simulink model "ADCS_Simulink"  (R2025b)
settings: Solver=FixedStepAuto  StartTime=0  StopTime=30  FixedStep=0.001  RelTol=1e-3
PreLoadFcn:
  | addpath(genpath('../'))
undefined symbols (not defined in the file or in its folder): DiscIntNeverNeededParam, IAU, juliandate
libraries: vrlib x16, simulink_extras x7, sharedtransform x5, sharedutil x4, aerolibutil x4, sFunctionLibrary x4, simulink x2, matrix_library x2, aerolibtransform2 x2
(part 2 of 2)

== matlab function ADCS_Simulink/Simulate Omega Rates/Wheel Torque ==
  data: wheel_speeds input; mag_bf input; GsValues input; L_R input; us output; tauMTB output; t_3axis output
function [us, tauMTB,t_3axis]  = f(wheel_speeds, mag_bf, GsValues, L_R)
% MATLAB Function block version of WheelTorque_Command
%
% Inputs:
%   wheel_speeds [4x1]   : Reaction wheel speeds [rad/s]
%   mag_bf       [3x1]   : Magnetic field vector in body frame [T]
%   GsValues     [3x4]   : Wheel geometry / spin axis matrix
%   L_R_input    [3x1]   : Desired control torque from PD controller [Nm]
%
% Output:
%   out_u [7x1] : [us(4x1); tauMTB(3x1)]

    % Constants
    Iws = 0.000029382450521;   % Wheel spin axis inertia [kg·m^2]
    c   = 0.025;                % Reaction wheel torque to magtorquer scaler
    OmegaD = rpm_to_rads(250) * ones(4,1);  % Desired wheel bias [rad/s]

    % Wheel speed vector
    Omega = wheel_speeds(:);

    % L_R from PD controller
    L_R = L_R(:);

    % Torque rod transformation (identity)
    Gt = eye(3);

    % Compute pseudo-inverse of Gs
    Gs = GsValues;
    Gs_pinv = pinv(Gs);

    % RW torque required to track commanded torque
    usReq = Gs_pinv * (-L_R);  %usReq is a 4 by 1 quantity

    % Despin torque
    usStar = -c * Iws * (Omega - OmegaD);

    % Skew-symmetric matrix of magnetic field
    B_tilde = [   0      -mag_bf(3)  mag_bf(2);
               mag_bf(3)     0      -mag_bf(1);
              -mag_bf(2)  mag_bf(1)     0     ];

     
    Btilde_Gt = B_tilde * Gt;
    muStar = -pinv(Btilde_Gt) * Gs * usStar;
    for i = 1:3
        if(muStar(i)>.1)
            muStar(i) = .1;
        end
        if(muStar(i)<-.1)
            muStar(i) = -.1;
        end
    end

    % Magnetic torque
    tauMTB = -(Btilde_Gt) * muStar;

    % deltaU = pinv(Gs) * (tauMTB - Gs*usStar)
    deltaU = Gs_pinv * (tauMTB - Gs * usStar);

    % Actual applied RW torque
    us = usReq + usStar + deltaU;

    for i = 1:4
        if(us(i)>.0032)
        us(i) = .0032;
        end
        if(us(i)<-.0032)
        us(i)=-.0032;
        end
    end

    t_3axis = -Gs*us;

end

% Helper: RPM to rad/s
function rad_s = rpm_to_rads(rpm)
    rad_s = rpm * (2*pi/60);
end

== matlab function ADCS_Simulink/Single Axis Error/Compute single axis rotation ==
  data: a input; y output; b input
function y = fcn(a, b)

axis = cross(a, b);
axis_norm = norm(axis);

if axis_norm < 1e-8
    if dot(a,b) > 0   %Vectors is parallel
        y = [1; 0; 0; 0];

    else              %Vectors are antiparallel
        axis = null(a(:).');
        axis = axis(:,1)/norm(axis(:,1));
        y = [0; axis];
    end
    return
end

axis = cross(a, b);
axis_norm = norm(axis);
axis = axis / axis_norm;
angle = acos(dot(a, b) / (norm(a)*norm(b)));

y = zeros(4,1);
y(1) = cos(angle / 2);
y(2:4) = axis * sin(angle / 2);

% if(y(1)<0)
%     y=-y;
% end

== matlab function ADCS_Simulink/Estimate Attitude/QUEST/MATLAB Function1 ==
  data: B_NED input; B_ECI output; lat input; lon input; JD input
function B_ECI = ned2eci(B_NED, lat, lon, JD)
% Converts magnetic field vector from NED to ECI
% Inputs:
%   B_NED = [Bn; Be; Bd] magnetic field vector in NED [any units]
%   lat, lon = geodetic latitude, longitude [deg]
%   JD = Julian Date
% Output:
%   B_ECI = [Bx; By; Bz] in ECI coordinates [same units]

lon = deg2rad(lon);
lat = deg2rad(lat);
% ----- 1. Compute GMST -----
JD0 = floor(JD + 0.5) - 0.5;
H = (JD - JD0) * 24;             % hours since 0h UT
D = JD - 2451545.0;
D0 = JD0 - 2451545.0;
T = D / 36525;

GMST_hours = 6.697374558 + 0.06570982441908 * D0 + 1.00273790935 * H + 0.000026 * T^2;
GMST_hours = mod(GMST_hours, 24);         % wrap 0-24h
theta_g = deg2rad(15 * GMST_hours);       % convert to radians

% ----- 2. Rotation from NED -> ECEF -----
R_ECEF_NED = [ -sin(lat)*cos(lon), -sin(lat)*sin(lon),  cos(lat);
               -sin(lon),            cos(lon),           0;
               -cos(lat)*cos(lon),  -cos(lat)*sin(lon), -sin(lat) ];

% ----- 3. Rotation from ECEF -> ECI -----
R_ECI_ECEF = [ cos(theta_g), -sin(theta_g), 0;
               sin(theta_g),  cos(theta_g), 0;
               0,              0,           1 ];

% ----- 4. Combine rotations -----
B_ECI = R_ECI_ECEF * R_ECEF_NED * B_NED;
end

== matlab function ADCS_Simulink/Simulate Omega Rates/Clamp WS ==
  data: u input; y output
function y = fcn(u)

max_threshold=6500*((2*pi)/60);
min_threshold=120*((2*pi)/60);

for i=1:4
if(u(i)>max_threshold)
    u(i)=max_threshold;
elseif(u(i)<-min_threshold)
    u(i)=-min_threshold;
end

end
y=u;

== matlab function ADCS_Simulink/Create Desired Quaternion/DCOMM & CSAC/MATLAB Function ==
  data: JD_now input; day output
function day = fcn(JD_now)

baseJD_start =  2.460950250000000e+06;
day = JD_now - baseJD_start;

== matlab function ADCS_Simulink/Angle Error1 ==
  data: u input; y output
function y = fcn(u)
    a = u(1);
    
    y = 2 * acos(a);
end

== matlab function ADCS_Simulink/Create Desired Quaternion/Check Flippage ==
  data: q input; y output
function y = fcn(q)

% persistent q_prev;
% if(isempty(q_prev))
%     q_prev=q;
% end
% 
% if(dot(q_prev,q)<0)
%     q=-q;
% end
% 
% q_prev=q;
% y=q;

if(q(1)<=0)
y=-q;
else
y=q;
end
end

== matlab function ADCS_Simulink/Estimate Attitude/QUEST/Sun_vec_eci ==
  data: sun_vec_eci output; decyear output; day output; t_utc input
function [sun_vec_eci, decyear, day] = SunVecECI_codegen(t_utc)
% Codegen-safe function for Simulink
% Input: t_utc (Julian Date)
% Outputs:
%   sun_vec_eci - 3x1 Sun unit vector in ECI
%   decyear     - decimal year (for IGRF)
%   day         - day of month (for IGRF)

% --- Constants ---
JD_J2000 = 2451545.0; % reference JD for 2000-01-01 12:00 UTC

% --- Compute approximate year ---
days_since_2000 = t_utc - JD_J2000;
year = 2000 + floor(days_since_2000 / 365.25);

% --- Compute day-of-year fraction ---
JD_start_of_year = JD_J2000 + (year-2000)*365.25; % approximate start of year
frac_day_of_year = t_utc - JD_start_of_year;

% --- Compute day of month (simplified for IGRF) ---
% approximate: 12 months = 365.25/12 ~ 30.4375 days per month
day = floor(mod(frac_day_of_year, 30.4375)) + 1;

% --- Decimal year ---
decyear = year + frac_day_of_year / 365.25;

% --- Clamp for IGRF ---
if decyear > 2025
    decyear = 2025;
elseif decyear < 1900
    decyear = 1900;
end

% --- Sun vector in ECI ---
D_days = t_utc - JD_J2000; % days since J2000
g = 357.529 + 0.98560028 * D_days;           
q = 280.459 + 0.98564736 * D_days;          
L = q + 1.914666471*sind(g) + 0.018994643*sind(2*g);
e = 23.439291 - 0.0130042*(D_days/36525); 

x = cosd(L);
y = cosd(e)*sind(L);
z = sind(e)*sind(L);
 sun_vec_eci = [x; y; z];
% sun_vec_eci= [-0.9672; 4; -0.10];

end

== matlab function ADCS_Simulink/Estimate Attitude/QUEST/Trace ==
  data: x input; y output
function y = fcn(x)

y=x(1,1)+x(2,2)+x(3,3);

== matlab function ADCS_Simulink/Angle Error2 ==
  data: u input; y output
function y = fcn(u)
    a = u(1);
    
    y = 2 * acos(a);
end

== matlab function ADCS_Simulink/Estimate Attitude/buildBk ==
  data: magVec input single; y output single size=[3 2]; sunVec input single
function y = combineMagSunMeas(magVec,sunVec)
    
    y = single(zeros(3,2));
    y(:,1) = magVec;
    y(:,2) = sunVec;
end

== matlab function ADCS_Simulink/Estimate Attitude/buildEci_k ==
  data: magVec input single; y output single size=[3 2]; sunVec input single
function y = combineMagSunMeas(magVec,sunVec)
    
    y = single(zeros(3,2));
    y(:,1) = magVec;
    y(:,2) = sunVec;
end

== matlab function ADCS_Simulink/Estimate Attitude/Angle Error2 ==
  data: u input; y output
function y = fcn(u)
    a = u(1);
    
    y = 2 * acos(a);
end

== matlab function ADCS_Simulink/Estimate Attitude/Check Flippage ==
  data: u input; y output
function y = fcn(u)

if u(1)<0
     y = -u;
else 
    y=u;
end

== matlab function ADCS_Simulink/Create Desired Quaternion/create DCM ==
  data: y output; dv input; v1 output; v2 output; vel input; doter output; var output
function [y,v1,v2,doter,var]  = fcn(dv,vel)
dv = -dv;
vel=vel/norm(vel);
unitx=[1; 0; 0];
unity=[0; 1; 0];


var=0;

crop=unitx;

doter=abs(dot(dv,crop));

if(doter<0.99)
v1=cross(dv,crop);

else %if parallel
var=1;
v1=cross(dv,unity);
end

v1=v1/norm(v1);
v2=cross(dv,v1);
v2=v2/norm(v2);

y=[dv,v1,v2];



end

== matlab function ADCS_Simulink/Create Desired Quaternion/DCOMM & CSAC/Determine best GS ==
  data: y output; pos_ecef input; bdangle output; best output
function [y, bdangle,best]= fcn(pos_ecef)

gnd_stat = [  -1286433.52, -4720122.48, 4079330.11;   % Ground Station 1 - Denver, USA
               3875201.89,   87312.44, 5025191.62;    % Ground Station 2 - London, UK
              -2476842.13,  4678921.75, -3556211.38;  % Ground Station 3 - Perth, Australia
               1112103.57, -6123457.23, 1210234.99 ]; % Ground Station 4 - Santiago, Chile

smallest = inf;
best=0;
bdangle=50;  %just a filler
for i=1:4
        gnd=gnd_stat(i,:);
  
        gs2sc=pos_ecef-gnd';
        distance=norm(gs2sc);
        zenrad=acos(dot(gs2sc,gnd)/(norm(gs2sc)*norm(gnd)));
        zenangle=rad2deg(zenrad);
       if zenangle<90
            if distance<smallest
                smallest=distance;
                best=i;
                bdangle=zenangle;
            end
       end
end
if best == 0
y=zeros(3,1);
% disp("Yo we got zeroes");
else
y=gnd_stat(best,:)';
end

== matlab function ADCS_Simulink/PD Controller/Calculate Error ==
  data: q1 input; q output; q2 input
function q = fcn(q1, q2)
% MATLAB IMPLEMENTATION

    w1 = q1(1); x1 = q1(2); y1 = q1(3); z1 = q1(4);
    w2 = q2(1); x2 = q2(2); y2 = q2(3); z2 = q2(4);

    w = w1*w2 - x1*x2 - y1*y2 - z1*z2;
    x = w1*x2 + x1*w2 + y1*z2 - z1*y2;
    y = w1*y2 - x1*z2 + y1*w2 + z1*x2;
    z = w1*z2 + x1*y2 - y1*x2 + z1*w2;

    q = [w; x; y; z];
    q=q/norm(q);

    % if(q(1)<0)
    %  q=-q;
    % end

% COPYING FLIGHT CODE

end

== matlab function ADCS_Simulink/Create Desired Quaternion/Mode Switch ==
  data: c input; y output; sv input; sc2gs input; phicone input; t input; dc input
function y = fcn(c,sv,sc2gs,phicone,t,dc)

% if(t>=200)
% c=3
% end
% if (t>400)
% c=2
% end

if c==1
y=sv;
elseif c==2
    if norm(dc)==0 
    y=sv;
    else
    y=sc2gs;
    end
elseif c==3
y=phicone;
else
y=sv;
end

== matlab function ADCS_Simulink/Calculate Desired Rates/Angle betwen 2 vec ==
  data: a input; y output; b input
function y = fcn(a,b)

val = dot(a,b)/(norm(a)*norm(b));
val = max(-1, min(1, val));
y = acos(val);

== matlab function ADCS_Simulink/Create Desired Quaternion/DCOMM & CSAC/final phicone vec ==
  data: svec input; y output; zenith input
function y = fcn(svec,zenith)

y = cosd(45)*zenith + sind(45)*svec;
y=y/norm(y);

== matlab function ADCS_Simulink/Simulate Omega Rates/Gravity Gradient Torque ==
  data: J input; Tgg output; pos_bf input
function Tgg = fcn(J, pos_bf)

mag=norm(pos_bf);
u_const=3.986004418e14;
u_bf=pos_bf/mag;


coef=3*u_const/(mag^3);
t1=J*u_bf;
init=cross(u_bf,t1);
Tgg=coef*init;
